simulink model "cell_model"  (R2022a)
settings: Solver=VariableStepAuto  StartTime=0.0  StopTime=sim_duration  FixedStep=simulation.setup.stepsize  RelTol=1e-3
undefined symbols (not defined in the file or in its folder): batt, cell_parameters
settings Model: Creator=Wenlin  LastModifiedBy=Wenlin

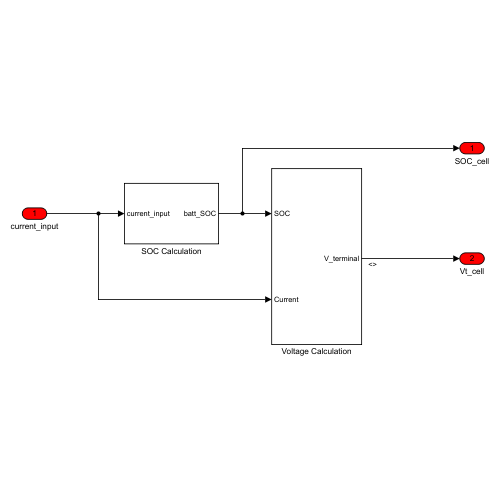
[thumbnail: Simulink's stored preview of the top-level diagram]
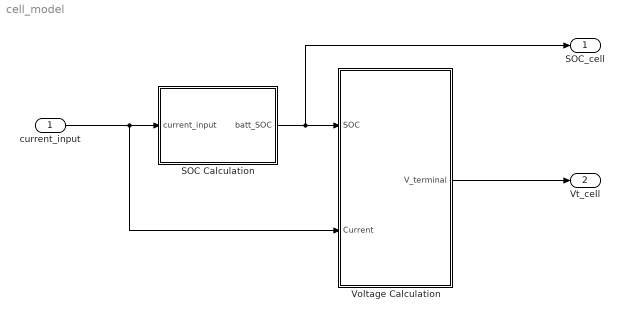
== system cell_model ==
  current_input : Inport
  SOC Calculation : Subsystem
  Voltage Calculation : Subsystem
  SOC_cell : Outport
  Vt_cell : Outport  Port=2
  wires:
  SOC Calculation/1(batt_SOC) -> SOC_cell/1, Voltage Calculation/1(SOC)
  current_input/1 -> Voltage Calculation/2(Current), SOC Calculation/1(current_input)
  Voltage Calculation/1(V_terminal) -> Vt_cell/1

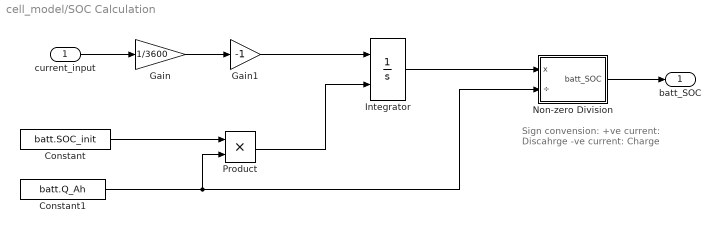
== system cell_model/SOC Calculation ==
  note: Sign convension:
      | +ve current: Discahrge
      | -ve current: Charge
  current_input : Inport
  Constant : Constant  Value=batt.SOC_init
  Constant1 : Constant  Value=batt.Q_Ah
  Gain : Gain  Gain=1/3600
  Gain1 : Gain  Gain=-1
  Integrator : Integrator  InitialConditionSource=external  InitialCondition=batt.SOC_init
  Non-zero Division : Subsystem
  Product : Product
  batt_SOC : Outport
  wires:
  Constant/1 -> Product/1
  Product/1 -> Integrator/2
  Gain/1 -> Gain1/1
  current_input/1 -> Gain/1
  Non-zero Division/1(batt_SOC) -> batt_SOC/1
  Constant1/1 -> Non-zero Division/2(÷), Product/2
  Integrator/1 -> Non-zero Division/1(x)
  Gain1/1 -> Integrator/1

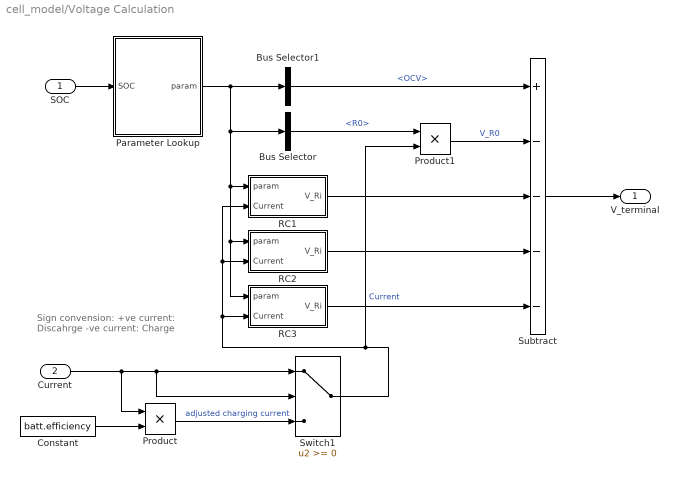
== system cell_model/Voltage Calculation ==
  note: Sign convension:
      | +ve current: Discahrge
      | -ve current: Charge
  SOC : Inport
  Current : Inport  Port=2
  Bus Selector : BusSelector  OutputSignals=R0
  Bus Selector1 : BusSelector  OutputSignals=OCV
  Constant : Constant  Value=batt.efficiency
  Parameter Lookup : Subsystem
  Product : Product
  Product1 : Product
  RC1 : Subsystem
  RC2 : Subsystem
  RC3 : Subsystem
  Subtract : Sum  Inputs=+----
  Switch1 : Switch  SaturateOnIntegerOverflow=off  InputSameDT=off
  V_terminal : Outport
  wires:
  SOC/1 -> Parameter Lookup/1(SOC)
  Bus Selector1/1 -> Subtract/1  "<OCV>"
  Product/1 -> Switch1/3  "adjusted charging current"
  Constant/1 -> Product/2
  Current/1 -> Switch1/1, Switch1/2, Product/1
  Switch1/1 -> RC3/2(Current), RC2/2(Current), RC1/2(Current), Product1/2  "Current"
  Product1/1 -> Subtract/2  "V_R0"
  Subtract/1 -> V_terminal/1
  Bus Selector/1 -> Product1/1  "<R0>"
  RC1/1(V_Ri) -> Subtract/3
  Parameter Lookup/1(param) -> RC3/1(param), RC2/1(param), RC1/1(param), Bus Selector/1, Bus Selector1/1
  RC2/1(V_Ri) -> Subtract/4
  RC3/1(V_Ri) -> Subtract/5

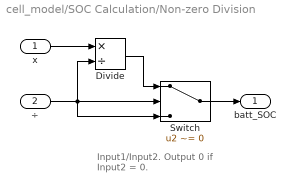
== system cell_model/SOC Calculation/Non-zero Division ==
  note: Input1/Input2.
      | Output 0 if Input2 = 0.
  x : Inport
  ÷ : Inport  Port=2
  Divide : Product  Inputs=*/
  Switch : Switch  Criteria=u2 ~= 0  SaturateOnIntegerOverflow=off  InputSameDT=off
  batt_SOC : Outport
  wires:
  ÷/1 -> Switch/2, Switch/3, Divide/2
  x/1 -> Divide/1
  Divide/1 -> Switch/1
  Switch/1 -> batt_SOC/1

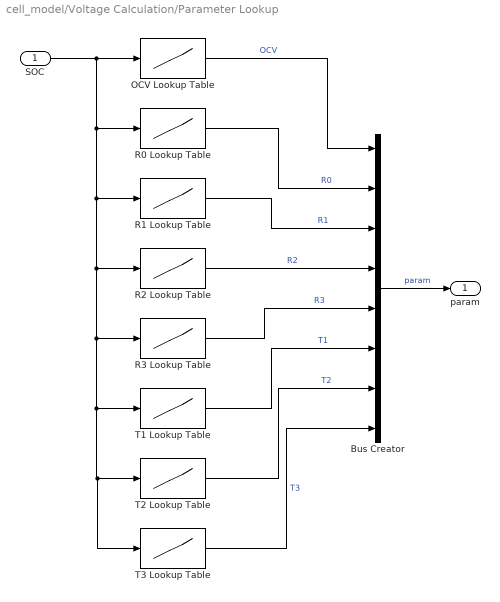
== system cell_model/Voltage Calculation/Parameter Lookup ==
  SOC : Inport
  Bus Creator : BusCreator  Inputs=8
  OCV Lookup Table : Lookup_n-D  NumberOfTableDimensions=1  BreakpointsForDimension1=cell_parameters.SOC  BreakpointsForDimension2=batt.elec_param.SOC  Table=cell_parameters.OCV  ExtrapMethod=Clip  UseLastTableValue=on  InternalRulePriority=Speed  RndMeth=Simplest
  R0 Lookup Table : Lookup_n-D  NumberOfTableDimensions=1  BreakpointsForDimension1=cell_parameters.SOC  BreakpointsForDimension2=batt.elec_param.SOC  Table=cell_parameters.R0  ExtrapMethod=Clip  UseLastTableValue=on  InternalRulePriority=Speed  RndMeth=Simplest
  R1 Lookup Table : Lookup_n-D  NumberOfTableDimensions=1  BreakpointsForDimension1=cell_parameters.SOC  BreakpointsForDimension2=batt.elec_param.SOC  Table=cell_parameters.RX(:, 1)  ExtrapMethod=Clip  UseLastTableValue=on  InternalRulePriority=Speed  RndMeth=Simplest
  R2 Lookup Table : Lookup_n-D  NumberOfTableDimensions=1  BreakpointsForDimension1=cell_parameters.SOC  BreakpointsForDimension2=batt.elec_param.SOC  Table=cell_parameters.RX(:, 2)  ExtrapMethod=Clip  UseLastTableValue=on  InternalRulePriority=Speed  RndMeth=Simplest
  R3 Lookup Table : Lookup_n-D  NumberOfTableDimensions=1  BreakpointsForDimension1=cell_parameters.SOC  BreakpointsForDimension2=batt.elec_param.SOC  Table=cell_parameters.RX(:, 3)  ExtrapMethod=Clip  UseLastTableValue=on  InternalRulePriority=Speed  RndMeth=Simplest
  T1 Lookup Table : Lookup_n-D  NumberOfTableDimensions=1  BreakpointsForDimension1=cell_parameters.SOC  BreakpointsForDimension2=batt.elec_param.SOC  Table=cell_parameters.TX(:, 1)  ExtrapMethod=Clip  UseLastTableValue=on  InternalRulePriority=Speed  RndMeth=Simplest
  T2 Lookup Table : Lookup_n-D  NumberOfTableDimensions=1  BreakpointsForDimension1=cell_parameters.SOC  BreakpointsForDimension2=batt.elec_param.SOC  Table=cell_parameters.TX(:, 2)  ExtrapMethod=Clip  UseLastTableValue=on  InternalRulePriority=Speed  RndMeth=Simplest
  T3 Lookup Table : Lookup_n-D  NumberOfTableDimensions=1  BreakpointsForDimension1=cell_parameters.SOC  BreakpointsForDimension2=batt.elec_param.SOC  Table=cell_parameters.TX(:, 3)  ExtrapMethod=Clip  UseLastTableValue=on  InternalRulePriority=Speed  RndMeth=Simplest
  param : Outport
  wires:
  Bus Creator/1 -> param/1  "param"
  R0 Lookup Table/1 -> Bus Creator/2  "R0"
  R1 Lookup Table/1 -> Bus Creator/3  "R1"
  R2 Lookup Table/1 -> Bus Creator/4  "R2"
  R3 Lookup Table/1 -> Bus Creator/5  "R3"
  T1 Lookup Table/1 -> Bus Creator/6  "T1"
  T2 Lookup Table/1 -> Bus Creator/7  "T2"
  T3 Lookup Table/1 -> Bus Creator/8  "T3"
  OCV Lookup Table/1 -> Bus Creator/1  "OCV"
  SOC/1 -> R1 Lookup Table/1, T3 Lookup Table/1, T2 Lookup Table/1, T1 Lookup Table/1, R3 Lookup Table/1, R2 Lookup Table/1, R0 Lookup Table/1, OCV Lookup Table/1

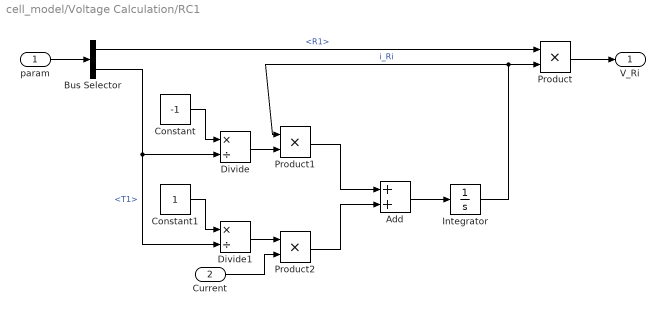
== system cell_model/Voltage Calculation/RC1 ==
  param : Inport
  Current : Inport  Port=2
  Add : Sum
  Bus Selector : BusSelector  OutputSignals=R1,T1
  Constant : Constant  Value=-1
  Constant1 : Constant
  Divide : Product  Inputs=*/
  Divide1 : Product  Inputs=*/
  Integrator : Integrator
  Product : Product
  Product1 : Product
  Product2 : Product
  V_Ri : Outport
  wires:
  Bus Selector/1 -> Product/1  "<R1>"
  Integrator/1 -> Product1/1, Product/2  "i_Ri"
  Product/1 -> V_Ri/1
  Add/1 -> Integrator/1
  Constant/1 -> Divide/1
  Divide/1 -> Product1/2
  Product1/1 -> Add/1
  Constant1/1 -> Divide1/1
  Bus Selector/2 -> Divide/2, Divide1/2  "<T1>"
  Divide1/1 -> Product2/1
  Current/1 -> Product2/2
  Product2/1 -> Add/2
  param/1 -> Bus Selector/1

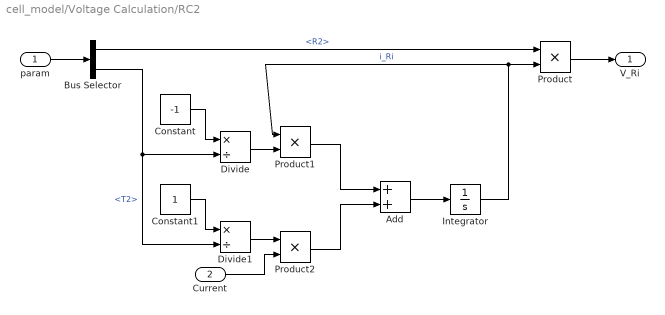
== system cell_model/Voltage Calculation/RC2 ==
  param : Inport
  Current : Inport  Port=2
  Add : Sum
  Bus Selector : BusSelector  OutputSignals=R2,T2
  Constant : Constant  Value=-1
  Constant1 : Constant
  Divide : Product  Inputs=*/
  Divide1 : Product  Inputs=*/
  Integrator : Integrator
  Product : Product
  Product1 : Product
  Product2 : Product
  V_Ri : Outport
  wires:
  param/1 -> Bus Selector/1
  Product2/1 -> Add/2
  Current/1 -> Product2/2
  Divide1/1 -> Product2/1
  Bus Selector/2 -> Divide1/2, Divide/2  "<T2>"
  Constant1/1 -> Divide1/1
  Product1/1 -> Add/1
  Divide/1 -> Product1/2
  Constant/1 -> Divide/1
  Add/1 -> Integrator/1
  Product/1 -> V_Ri/1
  Integrator/1 -> Product/2, Product1/1  "i_Ri"
  Bus Selector/1 -> Product/1  "<R2>"

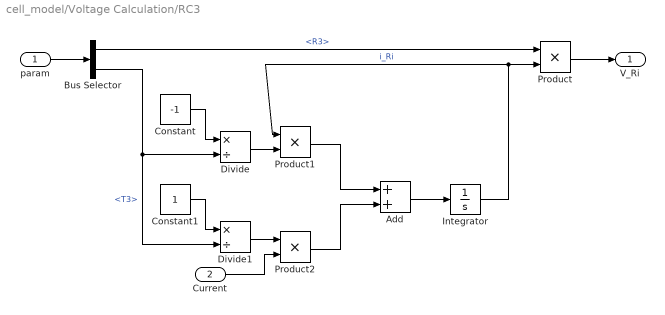
== system cell_model/Voltage Calculation/RC3 ==
  param : Inport
  Current : Inport  Port=2
  Add : Sum
  Bus Selector : BusSelector  OutputSignals=R3,T3
  Constant : Constant  Value=-1
  Constant1 : Constant
  Divide : Product  Inputs=*/
  Divide1 : Product  Inputs=*/
  Integrator : Integrator
  Product : Product
  Product1 : Product
  Product2 : Product
  V_Ri : Outport
  wires:
  Bus Selector/1 -> Product/1  "<R3>"
  Integrator/1 -> Product1/1, Product/2  "i_Ri"
  Product/1 -> V_Ri/1
  Add/1 -> Integrator/1
  Constant/1 -> Divide/1
  Divide/1 -> Product1/2
  Product1/1 -> Add/1
  Constant1/1 -> Divide1/1
  Bus Selector/2 -> Divide/2, Divide1/2  "<T3>"
  Divide1/1 -> Product2/1
  Current/1 -> Product2/2
  Product2/1 -> Add/2
  param/1 -> Bus Selector/1
